simulink model "c_caller"  (R2020b)
settings: Solver=FixedStepDiscrete  StartTime=0.0  StopTime=10.0  FixedStep=0.1  RelTol=1e-3  EnableMultiTasking=on
PostLoadFcn:
  | Simulink.importExternalCTypes(fullfile(matlabroot,'toolbox','simulink','simdemos','simfeatures','include','my_func.h'), 'EnumClass', 'dynamic');
undefined symbols (not defined in the file): TrafficLightColor
libraries: simulink x1
settings Model: Creator=The MathWorks, Inc.  LastModifiedBy=javier
settings DataIOCC: SaveFormat=StructureWithTime  SaveTime=off
settings OptimizationCC: DefaultParameterBehavior=Inlined  AccelVerboseBuild=on
settings DebuggingCC: ParameterTunabilityLossMsg=error  BusObjectLabelMismatch=none  PregeneratedLibrarySubsystemCodeDiagnostic=none  ArithmeticOperatorsInVariantConditions=warning
settings SFSimCC: SimCustomHeaderCode="#include \"my_func.h\""  SimUserSources=src/my_func.c  SimUserIncludeDirs=include  SimUseLocalCustomCode=off  SimAnalyzeCustomCode=on  MATLABDynamicMemAlloc=off
settings RTWCC: GenerateReport=on  RTWUseLocalCustomCode=off  RTWUseSimCustomCode=on  CustomHeaderCode="#include \"my_func.h\""  CustomInclude=include  CustomSource=src/my_func.c  LaunchReport=on
settings CodeAppCC: ForceParamTrailComments=on  OperatorAnnotations=on  StateflowObjectComments=on  MATLABSourceComments=on
settings GRTTargetCC: TargetLangStandard=C89/C90 (ANSI)  MatFileLogging=off
settings ConfigComp: CovMetricSettings=dw  CovSaveCumulativeToWorkspaceVar=on  CovSaveSingleToWorkspaceVar=on  CovExternalEMLEnable=off

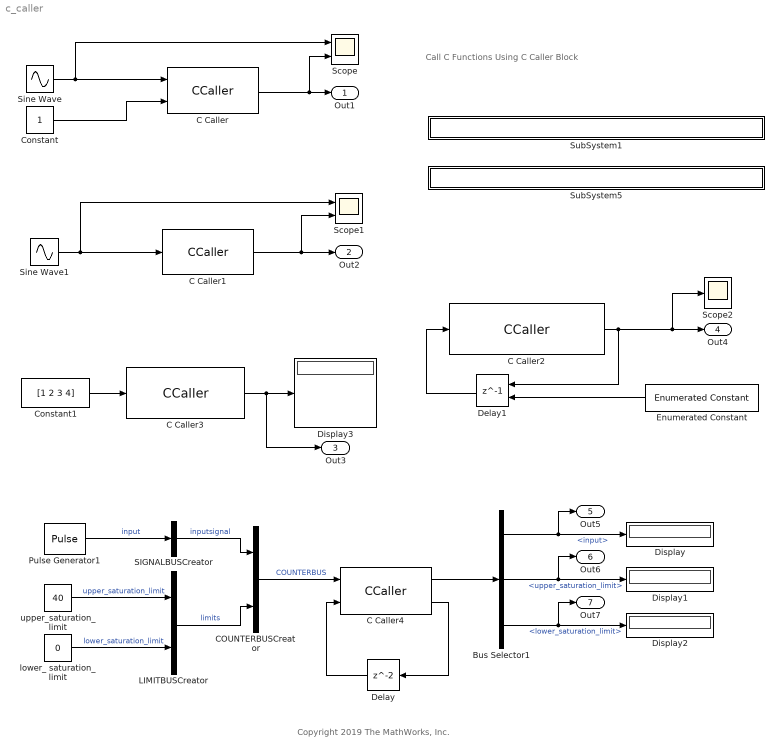
== system c_caller ==
  note: Copyright 2019 The MathWorks, Inc.
  note: Call C Functions Using C Caller Block
  Bus Selector1 : BusSelector  OutputSignals=inputsignal.input,limits.upper_saturation_limit,limits.lower_saturation_limit
  C Caller : CCaller  FunctionName=add  PortSpecificationStruct="%)30     .    6 4   8    (     @         %    \"     ,    !     0         %  0 \"0    $    _    07)G3F%M90  4&]R=$YA;64 4V-O<&4     26YD97@     5'EP90      4VEZ90      27-';&]B86P   X    P    !@    @    $          4    (     0    ,    !         !   P!O=70 #@   #     &    \"     0         !0    @    !     P    $         $  # &]U=  .    .     8    (    !          %    \"     $    &     0         0    !@   $]U='!U=   #@   #@    &    \"     8         !0    @    !     0    $         \"0    @               X    X    !@    @    $          4    (     0    8    !         !     &    9&]U8FQE   .    ,     8    (    !          %    \"     $    !     0         0  $ ,0    X    P    !@    @    ) @        4    (     0    $    !          (  0      #@   #     &    \"     0         !0    @    !     @    $         $  \" '4Q   .    ,     8    (    !          %    \"     $    \"     0         0  ( =3$   X    X    !@    @    $          4    (     0    4    !         !     %    26YP=70    .    .     8    (    !@         %    \"     $    !     0         )    \"               #@   #@    &    \"     0         !0    @    !    !@    $         $     8   !D;W5B;&4   X    P    !@    @    $          4    (     0    $    !         !   0 Q    #@   #     &    \"     D\"        !0    @    !     0    $          @ !       .    ,     8    (    !          %    \"     $    \"     0         0  ( =3(   X    P    !@    @    $          4    (     0    (    !         !   @!U,@  #@   #@    &    \"     0         !0    @    !    !0    $         $     4   !);G!U=     X    X    !@    @    &          4    (     0    $    !          D    (            \\#\\.    .     8    (    !          %    \"     $    &     0         0    !@   &1O=6)L90  #@   #     &    \"     0         !0    @    !     0    $         $  ! #$    .    ,     8    (    \"0(        %    \"     $    !     0         \"  $"
  C Caller1 : CCaller  FunctionName=timesK  PortSpecificationStruct="%)30     .    8 4   8    (     @         %    \"     ,    !     0         %  0 \"0    $    _    07)G3F%M90  4&]R=$YA;64 4V-O<&4     26YD97@     5'EP90      4VEZ90      27-';&]B86P   X    P    !@    @    $          4    (     0    ,    !         !   P!O=70 #@   #     &    \"     0         !0    @    !     P    $         $  # &]U=  .    .     8    (    !          %    \"     $    &     0         0    !@   $]U='!U=   #@   #@    &    \"     8         !0    @    !     0    $         \"0    @               X    X    !@    @    $          4    (     0    8    !         !     &    9&]U8FQE   .    ,     8    (    !          %    \"     $    !     0         0  $ ,0    X    P    !@    @    ) @        4    (     0    $    !          (  0      #@   #     &    \"     0         !0    @    !     0    $         $  ! '4    .    ,     8    (    !          %    \"     $    !     0         0  $ =0    X    X    !@    @    $          4    (     0    4    !         !     %    26YP=70    .    .     8    (    !@         %    \"     $    !     0         )    \"               #@   #@    &    \"     0         !0    @    !    !@    $         $     8   !D;W5B;&4   X    P    !@    @    $          4    (     0    $    !         !   0 Q    #@   #     &    \"     D\"        !0    @    !     0    $          @ !       .    ,     8    (    !          %    \"     $    !     0         0  $ 2P    X    P    !@    @    $          4    (     0    $    !         !   0!+    #@   $     &    \"     0         !0    @    !    \"0    $         $     D   !087)A;65T97(         #@   #@    &    \"     8         !0    @    !     0    $         \"0    @               X    X    !@    @    $          4    (     0    8    !         !     &    9&]U8FQE   .    ,     8    (    !          %    \"     $    !     0         0  $ ,0    X    P    !@    @    ) @        4    (     0    $    !          (  0"  K=2
  C Caller2 : CCaller  FunctionName=getNextTrafficLight  PortSpecificationStruct="%)30     .    Z ,   8    (     @         %    \"     (    !     0         %  0 \"0    $    _    07)G3F%M90  4&]R=$YA;64 4V-O<&4     26YD97@     5'EP90      4VEZ90      27-';&]B86P   X    P    !@    @    $          4    (     0    ,    !         !   P!O=70 #@   #     &    \"     0         !0    @    !     P    $         $  # &]U=  .    .     8    (    !          %    \"     $    &     0         0    !@   $]U='!U=   #@   #@    &    \"     8         !0    @    !     0    $         \"0    @               X   !(    !@    @    $          4    (     0   !<    !         !     7    16YU;3H@5')A9F9I8TQI9VAT0V]L;W( #@   #     &    \"     0         !0    @    !     0    $         $  ! #$    .    ,     8    (    \"0(        %    \"     $    !     0         \"  $       X    X    !@    @    $          4    (     0    <    !         !     '    8W5R<F5N=  .    .     8    (    !          %    \"     $    '     0         0    !P   &-U<G)E;G0 #@   #@    &    \"     0         !0    @    !    !0    $         $     4   !);G!U=     X    X    !@    @    &          4    (     0    $    !          D    (               .    2     8    (    !          %    \"     $    7     0         0    %P   $5N=6TZ(%1R869F:6-,:6=H=$-O;&]R  X    P    !@    @    $          4    (     0    $    !         !   0 Q    #@   #     &    \"     D\"        !0    @    !     0    $          @ !"
  C Caller3 : CCaller  FunctionName=incrementElement  PortSpecificationStruct="%)30     .    F 4   8    (     @         %    \"     ,    !     0         %  0 \"0    $    _    07)G3F%M90  4&]R=$YA;64 4V-O<&4     26YD97@     5'EP90      4VEZ90      27-';&]B86P   X    P    !@    @    $          4    (     0    $    !         !   0!U    #@   #     &    \"     0         !0    @    !     0    $         $  ! '4    .    0     8    (    !          %    \"     $    +     0         0    \"P   $EN<'5T3W5T<'5T       .    .     8    (    !@         %    \"     $    !     0         )    \"               #@   #@    &    \"     0         !0    @    !    !0    $         $     4   !I;G0S,@    X    P    !@    @    $          4    (     0    (    !         !   @ M,0  #@   #     &    \"     D\"        !0    @    !     0    $          @ !       .    ,     8    (    !          %    \"     $    $     0         0  0 <VEZ90X   !     !@    @    $          4    (     0    D    !         !     )    <VEZ92AU+#$I          X    X    !@    @    $          4    (     0    @    !         !     (    0V]N<W1A;G0.    .     8    (    !@         %    \"     $    !     0         )    \"               #@   #@    &    \"     0         !0    @    !    !@    $         $     8   !U:6YT,S(   X    P    !@    @    $          4    (     0    $    !         !   0 Q    #@   #     &    \"     D\"        !0    @    !     0    $          @ !       .    0     8    (    !          %    \"     $    -     0         0    #0   &EN8W)E;65N=%]I9'@    .    0     8    (    !          %    \"     $    -     0         0    #0   &EN8W)E;65N=%]I9'@    .    0     8    (    !          %    \"     $    )     0         0    \"0   %!A<F%M971E<@         .    .     8    (    !@         %    \"     $    !     0         )    \"            / _#@   #@    &    \"     0         !0    @    !    !@    $         $     8   !U:6YT,S(   X    P    !@    @    $          4    (     0    $    !         !   0 Q    #@   #     &    \"     D\"        !0    @    !     0    $          @ !"  increment_idx=uint32(1)
  C Caller4 : CCaller  FunctionName=counterbusFcn  PortSpecificationStruct="%)30     .    \" <   8    (     @         %    \"     0    !     0         %  0 \"0    $    _    07)G3F%M90  4&]R=$YA;64 4V-O<&4     26YD97@     5'EP90      4VEZ90      27-';&]B86P   X    P    !@    @    $          4    (     0    (    !         !   @!U,0  #@   #     &    \"     0         !0    @    !     @    $         $  \" '4Q   .    .     8    (    !          %    \"     $    %     0         0 ...(+2052 chars)"
  COUNTERBUSCreator : BusCreator  Inputs=2  OutDataTypeStr=Bus: COUNTERBUS  NonVirtualBus=on
  Constant : Constant
  Constant1 : Constant  Value=[1 2 3 4]  OutDataTypeStr=int32
  Delay : Delay
  Delay1 : Delay  DelayLength=1  InitialConditionSource=Input port
      settings: InputPortMap=u0,p4
  Display{,1..3} (4 alike) : Display
      Display settings: Format=short_e
      Display1 settings: Format=short_e
      Display2 settings: Format=short_e
  Enumerated Constant : simulink/Sources/Enumerated Constant  OutDataTypeStr=Enum: TrafficLightColor  Value=TrafficLightColor.GREEN  SampleTime=inf
  LIMITBUSCreator : BusCreator  Inputs=2  OutDataTypeStr=Bus: LIMITBUS  NonVirtualBus=on
  Pulse Generator1 : DiscretePulseGenerator  Amplitude=int32(1)  SampleTime=0.1
  SIGNALBUSCreator : BusCreator  Inputs=1  OutDataTypeStr=Bus: SIGNALBUS  NonVirtualBus=on
  Scope : Scope  NumInputPorts=2
  Scope1 : Scope  NumInputPorts=2
  Scope2 : Scope
  Sine Wave : Sin  SampleTime=0.1
  Sine Wave1 : Sin  SampleTime=0.1
  SubSystem1 : Subsystem  mask{filename=my_func.h}
      mask init:
      | x=sfundemo_maskdisp;
      settings: AttributesFormatString=\n  OpenFcn=sfundemo_openfcn
      mask Display: disp(x);
  SubSystem5 : Subsystem  mask{filename=my_func.c}
      mask init:
      | x=sfundemo_maskdisp;
      settings: AttributesFormatString=\n  OpenFcn=sfundemo_openfcn
      mask Display: disp(x);
  lower_ saturation_ limit : Constant  Value=0  OutDataTypeStr=int32
  upper_saturation_limit : Constant  Value=40  OutDataTypeStr=int32
  Out1 : Outport  VectorParamsAs1DForOutWhenUnconnected=off
  Out2 : Outport  Port=2  VectorParamsAs1DForOutWhenUnconnected=off
  Out3 : Outport  Port=3  VectorParamsAs1DForOutWhenUnconnected=off
  Out4 : Outport  Port=4  VectorParamsAs1DForOutWhenUnconnected=off
  Out5 : Outport  Port=5  VectorParamsAs1DForOutWhenUnconnected=off
  Out6 : Outport  Port=6  VectorParamsAs1DForOutWhenUnconnected=off
  Out7 : Outport  Port=7  VectorParamsAs1DForOutWhenUnconnected=off
  wires:
  Sine Wave/1 -> Scope/1, C Caller/1
  Constant/1 -> C Caller/2
  C Caller/1 -> Scope/2, Out1/1
  C Caller1/1 -> Out2/1, Scope1/2
  Sine Wave1/1 -> Scope1/1, C Caller1/1
  lower_ saturation_ limit/1 -> LIMITBUSCreator/2  "lower_saturation_limit"
  Bus Selector1/1 -> Out5/1, Display/1  "<input>"
  Bus Selector1/2 -> Display1/1, Out6/1  "<upper_saturation_limit>"
  C Caller4/1 -> Bus Selector1/1
  upper_saturation_limit/1 -> LIMITBUSCreator/1  "upper_saturation_limit"
  Delay/1 -> C Caller4/2
  COUNTERBUSCreator/1 -> C Caller4/1  "COUNTERBUS"
  Bus Selector1/3 -> Display2/1, Out7/1  "<lower_saturation_limit>"
  LIMITBUSCreator/1 -> COUNTERBUSCreator/2  "limits"
  C Caller4/2 -> Delay/1
  Pulse Generator1/1 -> SIGNALBUSCreator/1  "input"
  SIGNALBUSCreator/1 -> COUNTERBUSCreator/1  "inputsignal"
  C Caller2/1 -> Delay1/1, Out4/1, Scope2/1
  Delay1/1 -> C Caller2/1
  Enumerated Constant/1 -> Delay1/2
  C Caller3/1 -> Out3/1, Display3/1
  Constant1/1 -> C Caller3/1

== system c_caller/SubSystem1 ==

== system c_caller/SubSystem5 ==
